simulink model "SOAR_integration_test"  (R2018b)
settings: Solver=VariableStepAuto  StartTime=0.0  StopTime=10.0  RelTol=1e-3
undefined symbols (not defined in the file): FSW_Lib, fswParams
libraries: sharedutil x3, dspmtrx3 x2, MEKF_lib x2, aerolibutil x2, actuators_lib x1, CDH_command_lib x1, Environment_lib x1, Mekf_joseph x1, actuator_processing_lib x1, allocation_lib x1, control_command_generation_lib x1, evironmentEstimation_lib x1
(part 2 of 2)

== matlab function SOAR_integration_test/FSW_Lib/MEKF_lib/Subsystem Activated if: [All Sensors Valid] or [Gyro Bad and Sun//Mag sensors Valid]/TIME PROPAGATION of Q_EST, COVARIANCE/MATLAB Function11 ==
  data: Phi_discrete input; P_sq output; Q_sq input; P_sq input
function P_sq  = Cqr(Phi_discrete,Q_sq,P_sq)
%#codegen

C = [P_sq'*Phi_discrete';Q_sq'];
          [Tc,Uc] = qr(C);
%           Uc = full(Uc);
          sq_P_kp1 = Uc(1:6,1:6)';
%           P = sq_P_kp1'*sq_P_kp1;
          P_sq = sq_P_kp1;

== matlab function SOAR_integration_test/FSW_Lib/MEKF_lib/Subsystem Activated if: [Sun//Mag Sensor Invalid and Gyros are Valid] or [Gyro Invalid and Sun//Mag sensors Invalid]/TIME PROPAGATION of Q_EST, COVARIANCE/MATLAB Function9 ==
  data: omega input; omega_cross_matrix output
function omega_cross_matrix = makes_omega_cross_matrix(omega)

omega_cross_matrix = [0 -omega(3) omega(2);omega(3) 0 -omega(1);-omega(2) omega(1) 0];

== matlab function SOAR_integration_test/FSW_Lib/MEKF_lib/Subsystem Activated if: [All Sensors Valid] or [Gyro Bad and Sun//Mag sensors Valid]/TIME PROPAGATION of Q_EST, COVARIANCE/MATLAB Function ==
  data: omega_est input; om_mag output
function om_mag = om2_norm(omega_est)

om_mag = norm(omega_est);

== matlab function SOAR_integration_test/FSW_Lib/MEKF_lib/Subsystem Activated if: [All Sensors Valid] or [Gyro Bad and Sun//Mag sensors Valid]/TIME PROPAGATION of Q_EST, COVARIANCE/MATLAB Function2 ==
  data: u input; om_mag output
function om_mag = norm_check1(u)
%#codegen
if u == 0
    om_mag = 10^-10;
else
    om_mag = u;
end
end
